simulink model "three_DoF_aircraft_model"  (R2020a)
settings: Solver=VariableStepAuto  StartTime=0.0  StopTime=TF  RelTol=1e-3
values from neighbouring files (symbols this model uses):
  init_altitude = 2000    [initialise_constants.m]
  lat0 = deg2rad(21)    [initialise_constants.m]
  long0 = deg2rad(157)    [initialise_constants.m]
  x0 = [u_initial ... (first row only)    [initialise_constants.m]
undefined symbols (not defined in the file or in its folder): Earth, WGS84
libraries: simulink_extras x5, simulink x3, aerolibfltsims x2, aerolibatmos2 x1, aerolibactuator x1, aerolibtransform2 x1
settings Model: Creator=hwave  LastModifiedBy=hwave
settings DataIOCC: ExternalInput=getinputstruct(op_trim1)  InitialState=getstatestruct(op_trim1)  ReturnWorkspaceOutputs=off

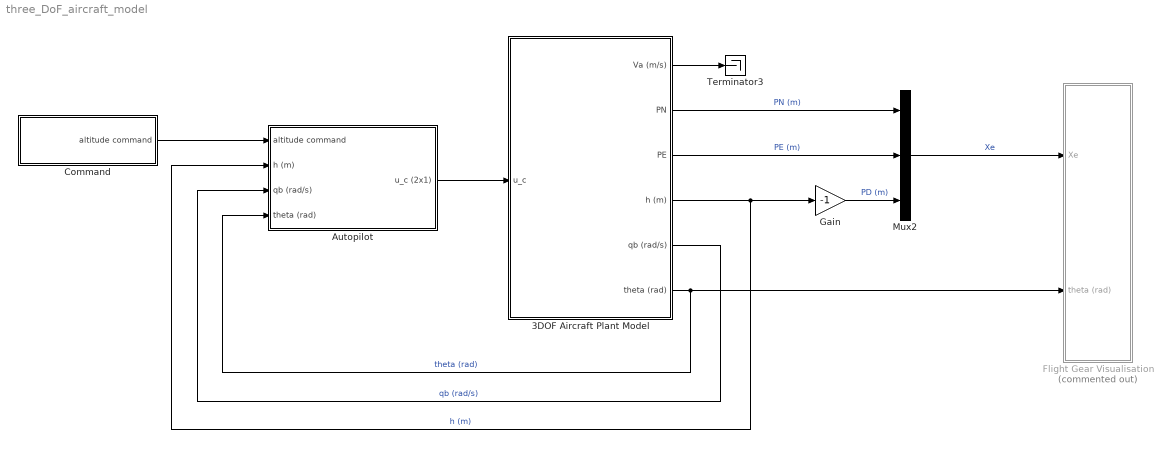
== system three_DoF_aircraft_model ==
  3DOF Aircraft Plant Model : Subsystem
  Autopilot : Subsystem
  Command : Subsystem
  Flight Gear Visualisation : Subsystem  Commented=on
  Gain : Gain  Gain=-1
  Mux2 : Mux  Inputs=3
  Terminator3 : Terminator
  wires:
  3DOF Aircraft Plant Model/6(theta (rad)) -> Flight Gear Visualisation/2(theta (rad)), Autopilot/4(theta (rad))  "theta (rad)"
  3DOF Aircraft Plant Model/4(h (m)) -> Gain/1, Autopilot/2(h (m))  "h (m)"
  3DOF Aircraft Plant Model/1(Va (m/s)) -> Terminator3/1
  3DOF Aircraft Plant Model/3(PE) -> Mux2/2  "PE (m)"
  3DOF Aircraft Plant Model/2(PN) -> Mux2/1  "PN (m)"
  Mux2/1 -> Flight Gear Visualisation/1(Xe)  "Xe"
  Gain/1 -> Mux2/3  "PD (m)"
  Command/1(altitude command) -> Autopilot/1(altitude command)
  3DOF Aircraft Plant Model/5(qb (rad/s)) -> Autopilot/3(qb (rad/s))  "qb (rad/s)"
  Autopilot/1(u_c (2x1)) -> 3DOF Aircraft Plant Model/1(u_c)

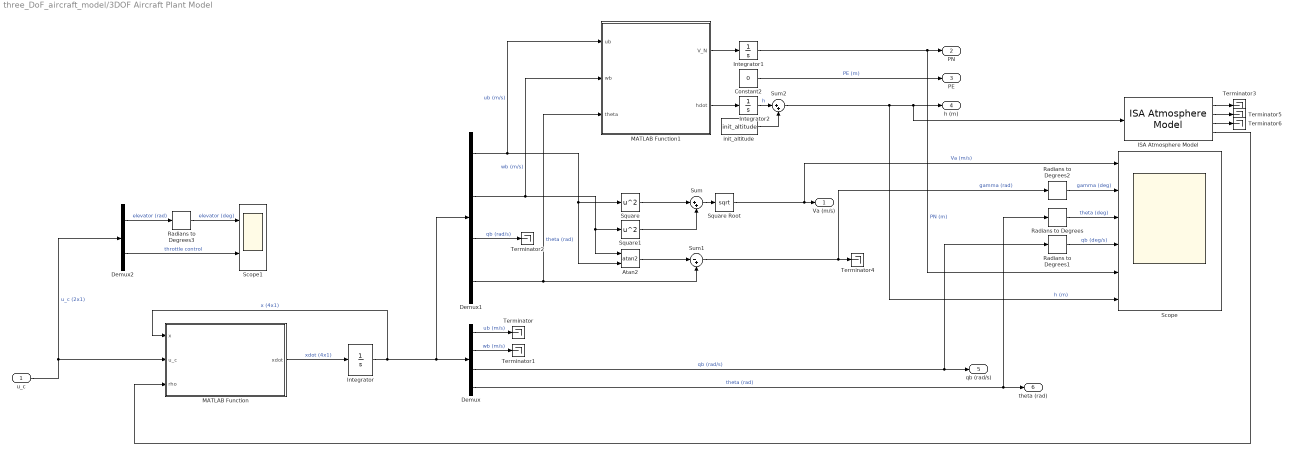
== system three_DoF_aircraft_model/3DOF Aircraft Plant Model ==
  u_c : Inport
  Atan2 : Trigonometry  Operator=atan2
  Constant2 : Constant  Value=0
  Demux : Demux
  Demux1 : Demux
  Demux2 : Demux  Outputs=2
  ISA Atmosphere Model : aerolibatmos2/ISA Atmosphere Model  custom=off  g=9.80665  gamma=1.4  R=287.0531  L=0.0065  h_trop=11000  h_strat=20000  rho0=1.225  P0=101325  T0=288.15  h0=0
  Integrator : Integrator  InitialCondition=x0
  Integrator1 : Integrator
  Integrator2 : Integrator
  MATLAB Function : MATLAB Function  TreatAsAtomicUnit=on
  MATLAB Function1 : MATLAB Function  TreatAsAtomicUnit=on
  Radians to Degrees{,1..3} (4 alike) : simulink_extras/Transformations/Radians to Degrees
  Scope : Scope  NumInputPorts=6
  Scope1 : Scope  NumInputPorts=2
  Square : Math  Operator=square  SaturateOnIntegerOverflow=on
  Square Root : Sqrt  SaturateOnIntegerOverflow=on
  Square1 : Math  Operator=square  SaturateOnIntegerOverflow=on
  Sum : Sum  Inputs=|++
  Sum1 : Sum  Inputs=|-+
  Sum2 : Sum  Inputs=|++
  Terminator{,1..6} (7 alike) : Terminator
  init_altitude : Constant  Value=init_altitude
  Va (m/s) : Outport
  PN : Outport  Port=2
  PE : Outport  Port=3
  h (m) : Outport  Port=4
  qb (rad/s) : Outport  Port=5
  theta (rad) : Outport  Port=6
  wires:
  MATLAB Function/1(xdot) -> Integrator/1  "xdot (4x1)"
  Integrator/1 -> Demux1/1, Demux/1, MATLAB Function/1(x)  "x (4x1)"
  Demux/4 -> Radians to Degrees/1, theta (rad)/1  "theta (rad)"
  Demux/3 -> Radians to Degrees1/1, qb (rad/s)/1  "qb (rad/s)"
  Demux/2 -> Terminator1/1  "wb (m/s)"
  Demux/1 -> Terminator/1  "ub (m/s)"
  Sum1/1 -> Radians to Degrees2/1, Terminator4/1  "gamma (rad)"
  Sum2/1 -> ISA Atmosphere Model/1, h (m)/1, Scope/6  "h (m)"
  Constant2/1 -> PE/1  "PE (m)"
  Integrator2/1 -> Sum2/1  "h"
  init_altitude/1 -> Sum2/2
  MATLAB Function1/1(V_N) -> Integrator1/1
  MATLAB Function1/2(hdot) -> Integrator2/1
  Integrator1/1 -> PN/1, Scope/5  "PN (m)"
  Square/1 -> Sum/1
  Demux1/2 -> MATLAB Function1/2(wb), Atan2/1, Square1/1  "wb (m/s)"
  Square Root/1 -> Scope/1, Va (m/s)/1  "Va (m/s)"
  Sum/1 -> Square Root/1
  Atan2/1 -> Sum1/1
  Demux1/4 -> MATLAB Function1/3(theta), Sum1/2  "theta (rad)"
  Demux1/1 -> MATLAB Function1/1(ub), Atan2/2, Square/1  "ub (m/s)"
  Square1/1 -> Sum/2
  Demux1/3 -> Terminator2/1  "qb (rad/s)"
  Demux2/2 -> Scope1/2  "throttle control"
  u_c/1 -> Demux2/1, MATLAB Function/2(u_c)  "u_c (2x1)"
  Radians to Degrees3/1 -> Scope1/1  "elevator (deg)"
  Demux2/1 -> Radians to Degrees3/1  "elevator (rad)"
  Radians to Degrees/1 -> Scope/3  "theta (deg)"
  Radians to Degrees1/1 -> Scope/4  "qb (deg/s)"
  Radians to Degrees2/1 -> Scope/2  "gamma (deg)"
  ISA Atmosphere Model/1 -> Terminator3/1
  ISA Atmosphere Model/2 -> Terminator5/1
  ISA Atmosphere Model/3 -> Terminator6/1
  ISA Atmosphere Model/4 -> MATLAB Function/3(rho)

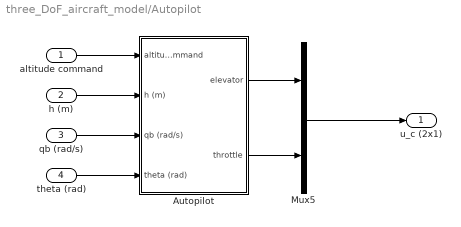
== system three_DoF_aircraft_model/Autopilot ==
  altitude command : Inport
  h (m) : Inport  Port=2
  qb (rad/s) : Inport  Port=3
  theta (rad) : Inport  Port=4
  Autopilot : Subsystem
  Mux5 : Mux  Inputs=2
  u_c (2x1) : Outport
  wires:
  Autopilot/1(elevator) -> Mux5/1
  Autopilot/2(throttle) -> Mux5/2
  Mux5/1 -> u_c (2x1)/1
  qb (rad/s)/1 -> Autopilot/3(qb (rad/s))
  theta (rad)/1 -> Autopilot/4(theta (rad))
  h (m)/1 -> Autopilot/2(h (m))
  altitude command/1 -> Autopilot/1(altitude command)

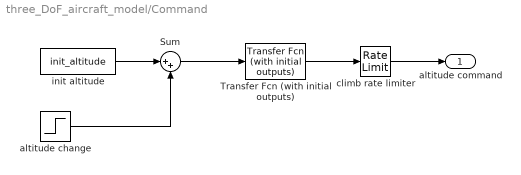
== system three_DoF_aircraft_model/Command ==
  Sum : Sum  Inputs=|++
  Transfer Fcn (with initial outputs) : simulink_extras/Additional Linear/Transfer Fcn (with initial outputs)  N=[0.25]  D="[1  0.25]"  Y0=init_altitude  U0=init_altitude
  altitude change : Step  Time=120  After=50  SampleTime=0
  climb rate limiter : RateLimiter  RisingSlewLimit=100/60  FallingSlewLimit=-100/60  SampleTimeMode=inherited  InitialCondition=init_altitude
  init altitude : Constant  Value=init_altitude  SampleTime=0
  altitude command : Outport
  wires:
  Transfer Fcn (with initial outputs)/1 -> climb rate limiter/1
  init altitude/1 -> Sum/1
  climb rate limiter/1 -> altitude command/1
  Sum/1 -> Transfer Fcn (with initial outputs)/1
  altitude change/1 -> Sum/2

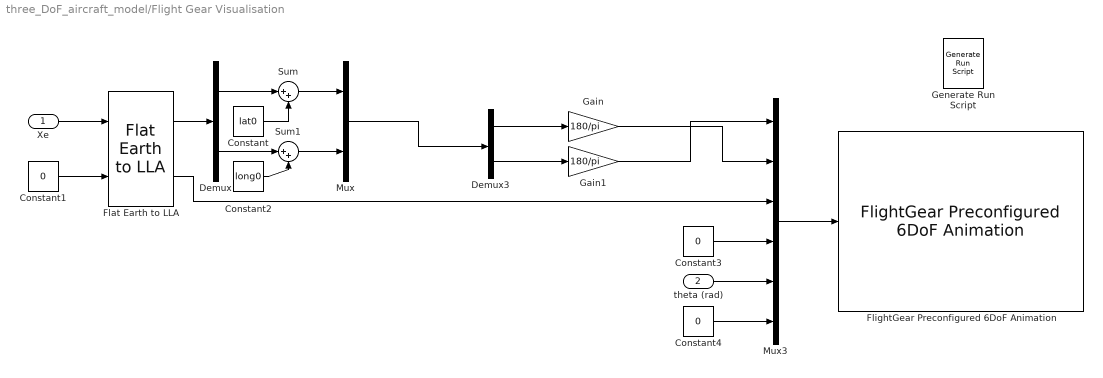
== system three_DoF_aircraft_model/Flight Gear Visualisation ==
  Xe : Inport
  theta (rad) : Inport  Port=2
  Constant : Constant  Value=lat0
  Constant1 : Constant  Value=0
  Constant2 : Constant  Value=long0
  Constant3 : Constant  Value=0
  Constant4 : Constant  Value=0
  Demux : Demux  Outputs=2
  Demux3 : Demux  Outputs=2
  Flat Earth to LLA : aerolibtransform2/Flat Earth to LLA  units=Metric (MKS)  ptype=Earth (WGS84)  F=1/298.257223563  R=6378137  refPosPort=off  LL0=[0 10]  psi=0
  FlightGear Preconfigured 6DoF Animation : aerolibfltsims/FlightGear Preconfigured 6DoF Animation  xFlightGearVersion=v2019.1  DestinationIpAddress=127.0.0.1  DestinationPort=5502  SampleTime=1/10  packetVersion=24
  Gain : Gain  Gain=180/pi
  Gain1 : Gain  Gain=180/pi
  Generate Run Script : aerolibfltsims/Generate Run Script  Architecture=Win64  dataFlow=Send  GeometryModelName=navion  AirportId=KSFO  RunwayId=10L  InitialAltitude=7224  InitialHeading=113  OffsetDistance=4.72  OffsetAzimuth=0  InstallScenery=on  DisableShaders=on  OriginAddress=127.0.0.1  DestinationPort=5502  OriginPort=5505  LocalAddress=127.0.0.1  OutputFileName=runfg.bat  FlightGearBaseDirectory=C:/Program Files/FlightGear 2019.1.1
  Mux : Mux  Inputs=2
  Mux3 : Mux  Inputs=6
  Sum : Sum  Inputs=|++
  Sum1 : Sum  Inputs=|++
  wires:
  Demux3/2 -> Gain1/1
  Constant1/1 -> Flat Earth to LLA/2
  Xe/1 -> Flat Earth to LLA/1
  Constant3/1 -> Mux3/4
  Gain/1 -> Mux3/2
  Flat Earth to LLA/2 -> Mux3/3
  Demux3/1 -> Gain/1
  Gain1/1 -> Mux3/1
  Mux3/1 -> FlightGear Preconfigured 6DoF Animation/1
  Constant4/1 -> Mux3/6
  Flat Earth to LLA/1 -> Demux/1
  theta (rad)/1 -> Mux3/5
  Demux/1 -> Sum/1
  Demux/2 -> Sum1/1
  Constant/1 -> Sum/2
  Constant2/1 -> Sum1/2
  Sum/1 -> Mux/1
  Sum1/1 -> Mux/2
  Mux/1 -> Demux3/1

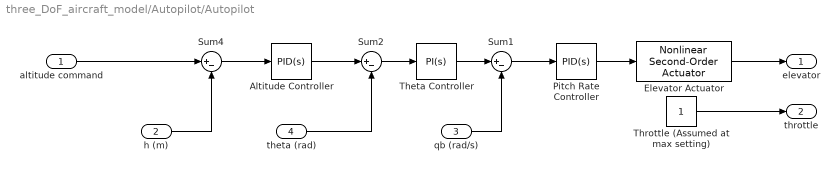
== system three_DoF_aircraft_model/Autopilot/Autopilot ==
  altitude command : Inport
  h (m) : Inport  Port=2
  qb (rad/s) : Inport  Port=3
  theta (rad) : Inport  Port=4
  Altitude Controller : simulink/Continuous/PID Controller  Controller=PID  Form=Parallel  TimeDomain=Continuous-time  UseExternalTs=off  SampleTime=-1  IntegratorMethod=Forward Euler  FilterMethod=Forward Euler  ControllerParametersSource=internal  P=0.0488507307473816  I=0.0131712663135505  D=0.0284455188618772  UseFilter=on  N=333.560229764619  TunerSelectOption=Transfer Function Based (PID Tuner App)  InitialConditionSource=internal  InitialConditionForIntegrator=0  InitialConditionForFilter=0  DifferentiatorICPrevScaledInput=0  ExternalReset=none  TrackingMode=off  Kt=1  LimitOutput=off  UpperSaturationLimit=inf  LowerSaturationLimit=-inf  LinearizeAsGain=on  AntiWindupMode=none  Kb=1  POutMin=[]  POutMax=[]  IOutMin=[]  IOutMax=[]  DOutMin=[]  DOutMax=[]  NOutMin=[]  NOutMax=[]  SumOutMin=[]  SumOutMax=[]  SaturationOutMin=[]  SaturationOutMax=[]  PParamMin=[]  PParamMax=[]  IParamMin=[]  IParamMax=[]  DParamMin=[]  DParamMax=[]  NParamMin=[]  NParamMax=[]  KbParamMin=[]  KbParamMax=[]  KtParamMin=[]  KtParamMax=[]  KbOutMin=[]  KbOutMax=[]  KtOutMin=[]  KtOutMax=[]  IntegratorOutMin=[]  IntegratorOutMax=[]  FilterOutMin=[]  FilterOutMax=[]  SumI1OutMin=[]  SumI1OutMax=[]  SumI2OutMin=[]  SumI2OutMax=[]  SumI3OutMin=[]  SumI3OutMax=[]  SumI4OutMin=[]  SumI4OutMax=[]  SumDOutMin=[]  SumDOutMax=[]  DifferentiatorOutMin=[]  DifferentiatorOutMax=[]  FilterDiffOutCoefMin=[]  FilterDiffOutCoefMax=[]  ReciprocalOutMin=[]  ReciprocalOutMax=[]  SumDenOutMin=[]  SumDenOutMax=[]  SumNumOutMin=[]  SumNumOutMax=[]  DivideOutMin=[]  DivideOutMax=[]  UdiffTsProdOutMin=[]  UdiffTsProdOutMax=[]  NTsProdOutMin=[]  NTsProdOutMax=[]  UintegralTsProdOutMin=[]  UintegralTsProdOutMax=[]  UngainTsProdOutMin=[]  UngainTsProdOutMax=[]  IntegratorContinuousStateAttributes=''  IntegratorStateMustResolveToSignalObject=off  IntegratorRTWStateStorageClass=Auto  FilterContinuousStateAttributes=''  FilterStateMustResolveToSignalObject=off  FilterRTWStateStorageClass=Auto  ParallelPVariant=InternalParameters  IdealPVariant=Disabled  IVariant=InternalParameters  DVariant=InternalParameters  IntegratorVariant=Continuous  SatVariant=Disabled  AWVariant=Passthrough  PCopyVariant=Disabled  TRVariant=Disabled  FdbkBlocksVariant=Forward  IdealPFdbkVariant=Disabled  SatFdbkVariant=Disabled  DerivativeFilterVariant=ContFilter  NVariant=InternalParameters  NCopyVariant=Disabled  FilterICVariant=InternalICsFilter  IntegratorICVariant=InternalICs  ExternalResetVariant=Disabled  TRSumVariant=Passthrough  SumFdbkVariant=Disabled  SumVariant=Sum_PID  TsampFilterVariant=InternalTs  TsampNgainVariant=Passthrough  TsampIntegralVariant=Passthrough
  Elevator Actuator : aerolibactuator/Nonlinear Second-Order Actuator  wn_fin=60  z_fin=0.7  fin_max=u_c1_max  fin_min=u_c1_min  fin_maxrate=180*pi/180  fin_act_0=0  fin_act_vel=0
      settings: SourceProductBaseCode=AE
  Pitch Rate Controller : simulink/Continuous/PID Controller  Controller=PID  Form=Parallel  TimeDomain=Continuous-time  UseExternalTs=off  SampleTime=-1  IntegratorMethod=Forward Euler  FilterMethod=Forward Euler  ControllerParametersSource=internal  P=-0.83865392873863  I=-10.8637077217053  D=-0.0159904694423334  UseFilter=on  N=3909.72848764398  TunerSelectOption=Transfer Function Based (PID Tuner App)  InitialConditionSource=internal  InitialConditionForIntegrator=0  InitialConditionForFilter=0  DifferentiatorICPrevScaledInput=0  ExternalReset=none  TrackingMode=off  Kt=1  LimitOutput=off  UpperSaturationLimit=inf  LowerSaturationLimit=-inf  LinearizeAsGain=on  AntiWindupMode=none  Kb=1  POutMin=[]  POutMax=[]  IOutMin=[]  IOutMax=[]  DOutMin=[]  DOutMax=[]  NOutMin=[]  NOutMax=[]  SumOutMin=[]  SumOutMax=[]  SaturationOutMin=[]  SaturationOutMax=[]  PParamMin=[]  PParamMax=[]  IParamMin=[]  IParamMax=[]  DParamMin=[]  DParamMax=[]  NParamMin=[]  NParamMax=[]  KbParamMin=[]  KbParamMax=[]  KtParamMin=[]  KtParamMax=[]  KbOutMin=[]  KbOutMax=[]  KtOutMin=[]  KtOutMax=[]  IntegratorOutMin=[]  IntegratorOutMax=[]  FilterOutMin=[]  FilterOutMax=[]  SumI1OutMin=[]  SumI1OutMax=[]  SumI2OutMin=[]  SumI2OutMax=[]  SumI3OutMin=[]  SumI3OutMax=[]  SumI4OutMin=[]  SumI4OutMax=[]  SumDOutMin=[]  SumDOutMax=[]  DifferentiatorOutMin=[]  DifferentiatorOutMax=[]  FilterDiffOutCoefMin=[]  FilterDiffOutCoefMax=[]  ReciprocalOutMin=[]  ReciprocalOutMax=[]  SumDenOutMin=[]  SumDenOutMax=[]  SumNumOutMin=[]  SumNumOutMax=[]  DivideOutMin=[]  DivideOutMax=[]  UdiffTsProdOutMin=[]  UdiffTsProdOutMax=[]  NTsProdOutMin=[]  NTsProdOutMax=[]  UintegralTsProdOutMin=[]  UintegralTsProdOutMax=[]  UngainTsProdOutMin=[]  UngainTsProdOutMax=[]  IntegratorContinuousStateAttributes=''  IntegratorStateMustResolveToSignalObject=off  IntegratorRTWStateStorageClass=Auto  FilterContinuousStateAttributes=''  FilterStateMustResolveToSignalObject=off  FilterRTWStateStorageClass=Auto  ParallelPVariant=InternalParameters  IdealPVariant=Disabled  IVariant=InternalParameters  DVariant=InternalParameters  IntegratorVariant=Continuous  SatVariant=Disabled  AWVariant=Passthrough  PCopyVariant=Disabled  TRVariant=Disabled  FdbkBlocksVariant=Forward  IdealPFdbkVariant=Disabled  SatFdbkVariant=Disabled  DerivativeFilterVariant=ContFilter  NVariant=InternalParameters  NCopyVariant=Disabled  FilterICVariant=InternalICsFilter  IntegratorICVariant=InternalICs  ExternalResetVariant=Disabled  TRSumVariant=Passthrough  SumFdbkVariant=Disabled  SumVariant=Sum_PID  TsampFilterVariant=InternalTs  TsampNgainVariant=Passthrough  TsampIntegralVariant=Passthrough
  Sum1 : Sum  Inputs=|+-
  Sum2 : Sum  Inputs=|+-
  Sum4 : Sum  Inputs=|+-
  Theta Controller : simulink/Continuous/PID Controller  Controller=PI  Form=Parallel  TimeDomain=Continuous-time  UseExternalTs=off  SampleTime=-1  IntegratorMethod=Forward Euler  FilterMethod=Forward Euler  ControllerParametersSource=internal  P=1.00231268426342  I=0.0172345719784472  D=0.257329571724935  UseFilter=on  N=28.9221873351667  TunerSelectOption=Transfer Function Based (PID Tuner App)  InitialConditionSource=internal  InitialConditionForIntegrator=0  InitialConditionForFilter=0  DifferentiatorICPrevScaledInput=0  ExternalReset=none  TrackingMode=off  Kt=1  LimitOutput=off  UpperSaturationLimit=inf  LowerSaturationLimit=-inf  LinearizeAsGain=on  AntiWindupMode=none  Kb=1  POutMin=[]  POutMax=[]  IOutMin=[]  IOutMax=[]  DOutMin=[]  DOutMax=[]  NOutMin=[]  NOutMax=[]  SumOutMin=[]  SumOutMax=[]  SaturationOutMin=[]  SaturationOutMax=[]  PParamMin=[]  PParamMax=[]  IParamMin=[]  IParamMax=[]  DParamMin=[]  DParamMax=[]  NParamMin=[]  NParamMax=[]  KbParamMin=[]  KbParamMax=[]  KtParamMin=[]  KtParamMax=[]  KbOutMin=[]  KbOutMax=[]  KtOutMin=[]  KtOutMax=[]  IntegratorOutMin=[]  IntegratorOutMax=[]  FilterOutMin=[]  FilterOutMax=[]  SumI1OutMin=[]  SumI1OutMax=[]  SumI2OutMin=[]  SumI2OutMax=[]  SumI3OutMin=[]  SumI3OutMax=[]  SumI4OutMin=[]  SumI4OutMax=[]  SumDOutMin=[]  SumDOutMax=[]  DifferentiatorOutMin=[]  DifferentiatorOutMax=[]  FilterDiffOutCoefMin=[]  FilterDiffOutCoefMax=[]  ReciprocalOutMin=[]  ReciprocalOutMax=[]  SumDenOutMin=[]  SumDenOutMax=[]  SumNumOutMin=[]  SumNumOutMax=[]  DivideOutMin=[]  DivideOutMax=[]  UdiffTsProdOutMin=[]  UdiffTsProdOutMax=[]  NTsProdOutMin=[]  NTsProdOutMax=[]  UintegralTsProdOutMin=[]  UintegralTsProdOutMax=[]  UngainTsProdOutMin=[]  UngainTsProdOutMax=[]  IntegratorContinuousStateAttributes=''  IntegratorStateMustResolveToSignalObject=off  IntegratorRTWStateStorageClass=Auto  FilterContinuousStateAttributes=''  FilterStateMustResolveToSignalObject=off  FilterRTWStateStorageClass=Auto  ParallelPVariant=InternalParameters  IdealPVariant=Disabled  IVariant=InternalParameters  DVariant=Disabled  IntegratorVariant=Continuous  SatVariant=Disabled  AWVariant=Passthrough  PCopyVariant=Disabled  TRVariant=Disabled  FdbkBlocksVariant=Forward  IdealPFdbkVariant=Disabled  SatFdbkVariant=Disabled  DerivativeFilterVariant=Disabled  NVariant=Disabled  NCopyVariant=Disabled_SignalSpec  FilterICVariant=Disabled  IntegratorICVariant=InternalICs  ExternalResetVariant=Disabled  TRSumVariant=Passthrough  SumFdbkVariant=Disabled  SumVariant=Sum_PI  TsampFilterVariant=InternalTs  TsampNgainVariant=Passthrough  TsampIntegralVariant=Passthrough
  Throttle (Assumed at max setting) : Constant
  elevator : Outport
  throttle : Outport  Port=2
  wires:
  Pitch Rate Controller/1 -> Elevator Actuator/1
  Sum4/1 -> Altitude Controller/1
  theta (rad)/1 -> Sum2/2
  Sum1/1 -> Pitch Rate Controller/1
  h (m)/1 -> Sum4/2
  Theta Controller/1 -> Sum1/1
  qb (rad/s)/1 -> Sum1/2
  Altitude Controller/1 -> Sum2/1
  Sum2/1 -> Theta Controller/1
  Elevator Actuator/1 -> elevator/1
  Throttle (Assumed at max setting)/1 -> throttle/1
  altitude command/1 -> Sum4/1

== matlab function three_DoF_aircraft_model/3DOF Aircraft Plant Model/MATLAB Function1 ==
  data: ub input; V_N output; wb input; theta input; hdot output
function [V_N, hdot] = navigation_equation(ub, wb, theta)

% This function is the longitudinal part of the navigation equations. It
% outputs velocity North, V_N and velocity down hdot.

velocity_vector_body = [ub; wb];

rotation_matrix = [cos(theta) -sin(theta);
                   sin(theta) cos(theta)];
               
velocity_vector_NED = rotation_matrix' * velocity_vector_body;

V_N = velocity_vector_NED(1);

% -ve value to ensure alignment with conventional axes system
hdot = -velocity_vector_NED(2);

== matlab function three_DoF_aircraft_model/3DOF Aircraft Plant Model/MATLAB Function ==
  data: x input; u_c input; xdot output; rho input
function xdot   = three_DoF_aircraft_simulator(x, u_c, rho)    

% By D. Clifford 28/08/2020

% A three degree of freedom aircraft simulator for integration with
% simulink. The aerodynamic model uses a vortex lattice method, using 7
% horseshoe vortices to model the aircraft; 4 for the wing; 1 for the
% stabiliser; 1 for the vertical stabiliser and 1 for the horizontal
% stabiliser. This model is only longitudinal, but adapating it to a 6
% degree of freedom simulator should be fairly trivial.

% Inputs are the state vector, x and control vector, u_c.

% The code also contains a short version of the navigation equations,
% calculating xe and ze. A more clear implementation of this is given in
% the Simulink model and so is commented out here.

% Some assumptions
% Lifting surfaces are modelled as thin, symmetrical flat plates. To
% account for camber, lookup the zero lift angle of attack, then add this
% to the wing setting angle in the aircraft_detail list. i.e. for the
% NACA 4412, the wing zero lift angle is -5 degrees. Therefore, positive 5
% degrees is added to the wing setting angle.
% The model only works under a small range of angles of attack. Stall and
% post stall conditions won't work at all here.

% NOTE
% Velocity is taken relative to the aircraft datum line, this means the
% force outputs, Fx and Fz are in the body axis

% NOTE
% See the initialise_constants script before running the Simulink model.

% extracting state vector terms
%xe = x(%);      % x position earth frame
%ze = x(%);      % z position earth frame +ve down
ub = x(1);      % aircraft body x velocity
wb = x(2);      % aircraft body z velocity
qb = x(3);      % aircraft body pitch rate
theta= x(4);    % aircraft body pitch angle

% extracting control vector terms
alpha_t = u_c(1);   % tail angle deflection
%throttle = u_c(2);  % throttle control

% initialising xdot
xdot = zeros(4, 1);

% initialising lists and matrices
xa = zeros(3, 7);
xb = zeros(3, 7);
xc = zeros(3, 7);
cc = zeros(3, 7);
n = zeros(3, 7);
Q = zeros(3, 7);
u = zeros(3, 7);
rhs = zeros(1, 7);
gamma = zeros(7, 1);
bc = zeros(3, 7);
A = zeros(7, 7);
Fx = zeros(1, 7);
Fz = zeros(1, 7);

%%%%%%%%%%%%%%%%%%%%%%%%%%%%%%%%%%%%%%%%%%%%%%%%%%%%%%%%%%%%%%%%%%%%%%%%%%%
%%%%%%%%%%%%%%%%%%%%%%%%%%% flight conditions %%%%%%%%%%%%%%%%%%%%%%%%%%%%%
%%%%%%%%%%%%%%%%%%%%%%%%%%%%%%%%%%%%%%%%%%%%%%%%%%%%%%%%%%%%%%%%%%%%%%%%%%%

Qinf = sqrt(ub^2 + wb^2);             % free stream velocity

% assuming the aircraft operates in altitudes close to sea level
%rho = 1.225;                          % free stream density
g = 9.81;                             % acc^ due to gravity

%%%%%%%%%%%%%%%%%%%%%%%%%%%%%%%%%%%%%%%%%%%%%%%%%%%%%%%%%%%%%%%%%%%%%%%%%%%
%%%%%%%%%%%%%%%%%%%%%%%%%%% navion specification %%%%%%%%%%%%%%%%%%%%%%%%%%
%%%%%%%%%%%%%%%%%%%%%%%%%%%%%%%%%%%%%%%%%%%%%%%%%%%%%%%%%%%%%%%%%%%%%%%%%%%

% specifications and flight conditions of a Navion found in
% "Aircraft Stability and Control Data" by G. L. Teper, April 1969
% all units have been converted to metric

% NOTE - approximations of certain geometric data have been made using the
% aircraft sketch given by G. L. Teper

% NOTE - Many of these dimensions and variables are not used due to the
% model's 3DOF restriction. Some dimensions such as dihedral angle are used
% but don't have a significant effect in this 3DOF model.

m = 1246.319;                         % aircraft mass
W = m * g;                            % aircraft total weight

lambda = -1;                          % engine, 0 for jet, -1 for piston
EP_HP = 200;                          % max engine power (horsepower)
EP_kW = EP_HP * 0.7457;               % max engine power kW
Ixx = 1421;
Iyy = 4068;
Izz = 4787;
Ixz = 0;

lw = -0.5;                            % dist from AC to cg
l = 5;                                % dist from wing AC to tailplane AC
lf = 2;                               % dist from fuselage front to wing AC

croot = 2.07384;                      % wing root chord
ctip = 1.20253;                       % wing tip chord
b_w = 10.18032;                       % wing span
S_w = ((croot + ctip) / 2)...         % wing planform area
       * 2 * b_w / 2;                 
AR_w = (b_w^2) / S_w;                 % wing aspect ratio
h0 = 0.25;                            % dist from wing LE to AC / by c_w

sweep_angle = 0 * pi / 180;           % wing sweep angle
dihedral_angle = 5 * pi / 180;        % wing dihedral angle
alpha_ws = 5 * pi / 180;              % wing setting angle

b_f = 1.4;                            % fuselage height
c_f = 8.1;                            % fuselage length
S_f  = b_f * c_f;                     % fuselage area
AR_f = (b_f^2) / S_f;                 % fuselage aspect ratio

c_tp_h = 1;                           % horizontal stabiliser chord
c_tp_v = 1.5;                         % vert stabiliser chord
AR_tp_h = 4;                          % horizontal stabiliser aspect ratio
AR_tp_v = 1;                          % vertical stabiliser aspect ratio

sigma = ctip / croot;                 % wing taper ratio
c_w = croot * (2 / 3) *...            % wing mean aerodynamic chord
      ((1 + sigma + sigma^2) /...
      (1 + sigma));   
b_tp_h = c_tp_h * AR_tp_h;            % horizontal stabiliser span
b_tp_v = c_tp_v * AR_tp_v;            % vertical stabiliser span              
S_tp_h = b_tp_h * c_tp_h;             % horizontal stabiliser span
S_tp_v = b_tp_v * c_tp_v;             % vertical stabiliser span

% an extremely rough approximation of total aircaft area (wetted area)
S_tot = S_w * 2 + S_f * 4 + S_tp_h + S_tp_v;

%%%%%%%%%%%%%%%%%%%%%%%%%%%%%%%%%%%%%%%%%%%%%%%%%%%%%%%%%%%%%%%%%%%%%%%%%%%
%%%%%%%%%%%%%%%%%%%%%%%% vortex geometry %%%%%%%%%%%%%%%%%%%%%%%%%%%%%%%%%%
%%%%%%%%%%%%%%%%%%%%%%%%%%%%%%%%%%%%%%%%%%%%%%%%%%%%%%%%%%%%%%%%%%%%%%%%%%%

lt = l - lw;                        % cg distance to tailplane ac
N_w = 4;                            % no. of main wing elements
N_tp_h = 1;                         % no. of horizontal tail plane elements
N_tp_v = 1;                         % no. vertical tail plane elements
N_f = 1;                            % no. of fuselage elements
Ntot = N_w + N_tp_h + N_tp_v + N_f; % total no. of vortex elements

% vortex element sizes
fact_w = sqrt(N_w / (N_w + 1));
fact_tp_h = sqrt(N_tp_h / (N_tp_h + 1));
fact_tp_v = sqrt(N_tp_v / (N_tp_v + 1));
fact_f = sqrt(N_f / (N_f + 1));

% length of the trailing vortices
large = 1.0e6;

% trailing vortex distance factors
bp = b_w * fact_w;
bp_f = b_f * fact_f;
dy = bp / N_w;
bp_tp_h = b_tp_h * fact_tp_h;
bp_tp_v = b_tp_v * fact_tp_h;

% control point to quarter chord dist
cp = 0.5 * c_w / fact_w;         % redefined after estabilish wing geometry
cp_f = 0.5 * c_f / fact_f;
cp_tp_h = 0.5 * c_tp_h / fact_tp_h;
cp_tp_v = 0.5 * c_tp_v / fact_tp_v;

%%%%%%%%%%%%%%%%%%%%%%%%%%%%%%%%%%%%%%%%%%%%%%%%%%%%%%%%%%%%%%%%%%%%%%%%%%%
%%%%%%%%%%%%%%%%%%%%%%%% wing vortex coordinates %%%%%%%%%%%%%%%%%%%%%%%%%%
%%%%%%%%%%%%%%%%%%%%%%%%%%%%%%%%%%%%%%%%%%%%%%%%%%%%%%%%%%%%%%%%%%%%%%%%%%%

% generates horseshoe vortex coordinates starting at the port wing tip and 
% ending at the starboard wing tip.

% port wing
xa(:, 1) = [(3 * dy / 2) * tan(sweep_angle);...
            2 * - dy;...
            (2 * dy / cos(sweep_angle)) * tan(dihedral_angle)];
xb(:, 1) = [(3 * dy / 2) * tan(sweep_angle);...
            - dy;...
            (dy / cos(sweep_angle)) * tan(dihedral_angle)];
xa(:, 2) = xb(:, 1) - [dy * tan(sweep_angle); 0; 0];
xb(:, 2) = xa(:, 2) + [0.0;...
                       dy;...
                       - (dy / cos(sweep_angle)) * tan(dihedral_angle)];
                   
% starboard wing
xa(:, 3) = [(dy / 2) * tan(sweep_angle); 0.0; 0.0];
xb(:, 3) = [(dy / 2) * tan(sweep_angle);...
            dy;...
            (dy / cos(sweep_angle)) * tan(dihedral_angle)];
xa(:, 4) = xb(:, 3) + [dy * tan(sweep_angle); 0; 0];
xb(:, 4) = xa(:, 4) + [0.0;...
                       dy;...
                       (dy / cos(sweep_angle)) * tan(dihedral_angle)];

% coords of centre of horseshoe vortices
cc(:, :) = 0.5 * (xa(:, :) + xb(:, :));

% assigning wing coords to horseshoe vortices using the local chord for a
% straight tapered wing equation
cw = croot + (2 * abs(cc(2, :)) / b_w) * (ctip - croot);

% control point distance factors
cp = 0.5 * cw / fact_w;

% wing control point locations and normal vectors
for i = 1 : 4
    xc(:, i) = 0.5 * (xa(:, i) + xb(:, i)) +...
               [cos(alpha_ws) * cp(i); 0.0; sin(alpha_ws) * cp(i)];
end

% port wing normal vectors
L1 = xb(:, 1) - xa(:, 1);
L2 = xc(:, 1) - xa(:, 1);

norm1 = cross(L1, L2);
mag1 = sqrt(norm1(1)^2+norm1(2)^2+norm1(3)^2);
unitnorm1 = norm1 / mag1;

n(:, 1) = unitnorm1 * -1;
n(:, 2) = unitnorm1 * -1;

% starboard wing normal vectors
L3 = xb(:, 3) - xa(:, 3);
L4 = xc(:, 3) - xa(:, 3);

norm2 = cross(L3, L4);
mag2 = sqrt(norm2(1)^2+norm2(2)^2+norm2(3)^2);
unitnorm2 = norm2 / mag2;

n(:, 3) = unitnorm2 * -1;
n(:, 4) = unitnorm2 * -1;


%%%%%%%%%%%%%%%%%%%%%%%%%%%%%%%%%%%%%%%%%%%%%%%%%%%%%%%%%%%%%%%%%%%%%%%%%%%
%%%%%%%%%%%%%%%%% horizontal stabiliser vortex coordinates %%%%%%%%%%%%%%%%
%%%%%%%%%%%%%%%%%%%%%%%%%%%%%%%%%%%%%%%%%%%%%%%%%%%%%%%%%%%%%%%%%%%%%%%%%%%

% coordinates of vortex segment on horizontal stabiliser
xa(:, 5) = [l; - 0.5 * bp_tp_h; 0.0];
xb(:, 5) = [l; + 0.5 * bp_tp_h; 0.0];
xc(:, 5) = 0.5 * (xa(:, 5) + xb(:, 5)) +...
                 [cos(alpha_t) * cp_tp_h; 0; sin(alpha_t) * cp_tp_h];

% tail plane normal vector
n(:, 5) = [sin(alpha_t); 0.0; cos(alpha_t)];

%%%%%%%%%%%%%%%%%%%%%%%%%%%%%%%%%%%%%%%%%%%%%%%%%%%%%%%%%%%%%%%%%%%%%%%%%%%
%%%%%%%%%%%%%%%%% vertical stabiliser vortex coordinates %%%%%%%%%%%%%%%%%%
%%%%%%%%%%%%%%%%%%%%%%%%%%%%%%%%%%%%%%%%%%%%%%%%%%%%%%%%%%%%%%%%%%%%%%%%%%%

% coordinates of vortex segment on vertical stabiliser
xa(:, 6) = [l; 0.0; 0.0];
xb(:, 6) = [l; 0.0; bp_tp_v];
xc(:, 6) = 0.5 * (xa(:, 6) + xb(:, 6)) +...
                 [cp_tp_v; 0.0; 0.0];

% tail plane normal vector
n(:, 6) = [0.0; 1.0; 0.0];

%%%%%%%%%%%%%%%%%%%%%%%%%%%%%%%%%%%%%%%%%%%%%%%%%%%%%%%%%%%%%%%%%%%%%%%%%%%
%%%%%%%%%%%%%%%%%%%%% fuselage vortex coordinates %%%%%%%%%%%%%%%%%%%%%%%%%
%%%%%%%%%%%%%%%%%%%%%%%%%%%%%%%%%%%%%%%%%%%%%%%%%%%%%%%%%%%%%%%%%%%%%%%%%%%

% coordinates of vortex segment on fuselage
xa(:, 7) = [-lf; 0.0; -bp_f];
xb(:, 7) = [-lf; 0.0; 0.0];
xc(:, 7) = 0.5 * (xa(:, 7) + xb(:, 7)) + [cp_f; 0.0; 0.0];

% fuselage normal vector
n(:, 7) = [0.0; 1.0; 0.0];

% velocity vectors (relative to the aircraft datum line)
% wing panels from port wing tip to starboard wing tip
Q(:, 1) = [ub + (qb * (-3 * dy / 2 * (cos(sweep_angle))) * tan(dihedral_angle));...
           0.0;...
           wb - (qb * (-(cp(1) - (lw - (3 * dy / 2) * tan(sweep_angle)))))];

Q(:, 2) = [ub + (qb * (-dy / 2 *(cos(sweep_angle))) * tan(dihedral_angle));...
           0.0;...
           wb - (qb * (-(cp(2) - (lw - (dy / 2) * tan(sweep_angle)))))];

Q(:, 3) = [ub + (qb * (-dy / 2 *(cos(sweep_angle))) * tan(dihedral_angle));...
           0.0;...
           wb - (qb * (-(cp(3) - (lw - (dy / 2) * tan(sweep_angle)))))];
       
Q(:, 4) = [ub + (qb * (-3 * dy / 2 *(cos(sweep_angle))) * tan(dihedral_angle));...
           0.0;...
           wb - (qb * (-(cp(4) - (lw - (3 * dy / 2) * tan(sweep_angle)))))];
       
% horizontal stabiliser
Q(:, 5) = [ub; 0.0; wb - qb * (-lt - cp_tp_h)]; 

% vertical stabiliser
Q(:, 6) = [ub + (qb * (-bp_tp_v / 2)); 0.0; wb - (qb * (-lt - cp_tp_v))];

% fuselage
Q(:, 7) = [ub + (qb * (bp_f / 2)); 0.0; wb - (qb * (-(cp_f - (lf + lw))))];

%%%%%%%%%%%%%%%%%%%%%%%%%%%%%%%%%%%%%%%%%%%%%%%%%%%%%%%%%%%%%%%%%%%%%%%%%%%
%%%%%%%%%%%%%%%%%%%%% solving circulation matrix %%%%%%%%%%%%%%%%%%%%%%%%%%
%%%%%%%%%%%%%%%%%%%%%%%%%%%%%%%%%%%%%%%%%%%%%%%%%%%%%%%%%%%%%%%%%%%%%%%%%%%
       
% set matrix and right hand side elements and solve for circulations
for i = 1 : 7
    for j = 1 : 7
        I = vfil(xa(:, j), xb(:, j), xc(:, i));
        I = I + vfil(xa(:, j) + [large; 0; 0], xa(:, j), xc(:, i));
        I = I + vfil(xb(:, j), xb(:, j) + [large; 0; 0], xc(:, i));
        A(i, j) = I(1) * n(1, i) + I(2) * n(2, i) + I(3) * n(3, i);
    end
    rhs(i)= - (Q(1, i) * n(1, i) + Q(2, i) * n(2, i) + Q(3, i) * n(3,i));
end

% solved circulation
gamma = A \ rhs';

%%%%%%%%%%%%%%%%%%%%%%%%%%%%%%%%%%%%%%%%%%%%%%%%%%%%%%%%%%%%%%%%%%%%%%%%%%%
%%%%%%%%%%%%%%%%%%% calculating forces and local velocity %%%%%%%%%%%%%%%%%
%%%%%%%%%%%%%%%%%%%%%%%%%%%%%%%%%%%%%%%%%%%%%%%%%%%%%%%%%%%%%%%%%%%%%%%%%%%

% force at centre of bound vortices
bc(:, :) = 0.5 * (xa(:, :) + xb(:, :));

% velocity vectors (relative to the aircraft datum line)
% wing panels from port wing tip to starboard wing tip
Q(:, 1) = [ub + (qb * (-3 * dy / 2 *(cos(sweep_angle))) * tan(dihedral_angle));...
           0.0;...
           wb - (qb * (-(- (lw - (3 * dy / 2) * tan(sweep_angle)))))];

Q(:, 2) = [ub + (qb * (-dy / 2 *(cos(sweep_angle))) * tan(dihedral_angle));...
           0.0;...
           wb - (qb * (-(- (lw - (dy / 2) * tan(sweep_angle)))))];

Q(:, 3) = [ub + (qb * (-dy / 2 *(cos(sweep_angle))) * tan(dihedral_angle));...
           0.0;...
           wb - (qb * (-(- (lw - (dy / 2) * tan(sweep_angle)))))];
       
Q(:, 4) = [ub + (qb * (-3 * dy / 2 *(cos(sweep_angle))) * tan(dihedral_angle));...
           0.0;...
           wb - (qb * (-(- (lw - (3 * dy / 2) * tan(sweep_angle)))))];
       
% horizontal stabiliser
Q(:, 5) = [ub; 0.0; wb - qb * (-lt)]; 

% vertical stabiliser
Q(:, 6) = [ub + (qb * (-bp_tp_v / 2)); 0.0; wb - (qb * (-lt))];

% fuselage
Q(:, 7) = [ub + (qb * (bp_f / 2)); 0.0; wb - (qb * (-(- (lf + lw))))];

for i = 1 : 7
    % finding the local velocity vector u on each load element i
    u(:, i) = Q (:, i);
    for j = 1 : 7
        u(:, i) = u(:, i) + vfil(xa(:, j), xb(:, j), bc(:, i)) * gamma(j);
        u(:, i) = u(:, i) + vfil(xa(:, j) +...
                  [large;0;0], xa(:,j), bc(:,i)) * gamma(j);
        u(:, i) = u(:, i) + vfil(xb(:, j), xb(:,j) +...
                  [large;0;0], bc(:,i)) * gamma(j);
    end
    % u cross s gives the direction of the force
    s = xb(:, i) - xa(:, i);
    Fx(i) = rho * (u(2, i) * s(3) - u(3, i) * s(2)) * gamma(i);
    Fz(i) = rho * (u(1, i) * s(2) - u(2, i) * s(1)) * gamma(i);
end

%%%%%%%%%%%%%%%%%%%%%%%%%%%%%%%%%%%%%%%%%%%%%%%%%%%%%%%%%%%%%%%%%%%%%%%%%%%
%%%%%%%%%%%%%%%% zero lift drag coefficient estimate %%%%%%%%%%%%%%%%%%%%%%
%%%%%%%%%%%%%%%%%%%%%%%%%%%%%%%%%%%%%%%%%%%%%%%%%%%%%%%%%%%%%%%%%%%%%%%%%%%

% viscosity of air at sea level
mu = 1.789e-5;

% reynolds number
Re_w = (rho * Qinf * (S_tot/b_w))/mu;

% skin friction coefficient 
Cfe_w = 0.00258 + 0.00102 * exp((-6.28e-9) * Re_w) +...
       0.00295 * exp((-2.01e-8) * Re_w);
   
% calculating zero lift drag coefficient
CD0 = Cfe_w * (S_tot/S_w);

% calculating zero lift drag
d0_w = CD0 * 0.5 * rho * Qinf^2 * S_w;
d0_tp_h = CD0 * (S_tp_h / S_w) * 0.5 * rho * Qinf^2 * S_tp_h;
d0_tp_v = CD0 * (S_tp_v / S_w) * 0.5 * rho * Qinf^2 * S_tp_v;
d0_f = CD0 * (S_f / S_w) * 0.5 * rho * Qinf^2 * S_f;

%%%%%%%%%%%%%%%%%%%%%%%%%%%%%%%%%%%%%%%%%%%%%%%%%%%%%%%%%%%%%%%%%%%%%%%%%%%
%%%%%%%%%%%%%%%%%%%%%%%%%%%% outputs %%%%%%%%%%%%%%%%%%%%%%%%%%%%%%%%%%%%%%
%%%%%%%%%%%%%%%%%%%%%%%%%%%%%%%%%%%%%%%%%%%%%%%%%%%%%%%%%%%%%%%%%%%%%%%%%%%

% pitching moment about aircraft cg
M = Fz(1) * (lw - bc(1, 1)) + Fz(2) * (lw - bc(1, 2)) +...
    Fz(3) * (lw - bc(1, 3)) + Fz(4) * (lw - bc(1, 4)) -...
    Fz(5) * lt;

% total z body force
Fzb = sum(Fz(1:Ntot));

% total x body force
Fxb = sum(Fx(1:Ntot)) + d0_w + d0_tp_h + d0_tp_v + d0_f;

%%%%%%%%%%%%%%%%%%%%%%%%%%%%%%%%%%%%%%%%%%%%%%%%%%%%%%%%%%%%%%%%%%%%%%%%%%%
%%%%%%%%%%%%%%%%%%%%%%%%%%%%% thrust calculation %%%%%%%%%%%%%%%%%%%%%%%%%%
%%%%%%%%%%%%%%%%%%%%%%%%%%%%%%%%%%%%%%%%%%%%%%%%%%%%%%%%%%%%%%%%%%%%%%%%%%%

% thrust
thrust = EP_kW * 1000 / sqrt(ub^2 + wb^2);

%%%%%%%%%%%%%%%%%%%%%%%%%%%%%%%%%%%%%%%%%%%%%%%%%%%%%%%%%%%%%%%%%%%%%%%%%%%
%%%%%%%%%%%%%%%%%%%%%%%%%%%%% state vector %%%%%%%%%%%%%%%%%%%%%%%%%%%%%%%%
%%%%%%%%%%%%%%%%%%%%%%%%%%%%%%%%%%%%%%%%%%%%%%%%%%%%%%%%%%%%%%%%%%%%%%%%%%%

% align forces with correct axis directions
Fxbr = - Fxb;
Fzbr = - Fzb;

% adding thrust component to x body force
Fxbr = Fxbr + u_c(2) * thrust - W * sin(theta);
Fzbr = Fzbr + W * cos(theta);

% location in earth reference frame
%xdot(1) = cos(theta) * ub + sin(theta) * wb;
%xdot(2)= -sin(theta) * ub + cos(theta) * wb;

xdot(1) = (Fxbr / m) - (qb * wb);
xdot(2) = (Fzbr / m) + (qb * ub);

xdot(3) = M / Iyy;

xdot(4)= qb;


end
